simulink model "ADRC_2X2_decoupling"  (Simulink 7.6)
settings: Solver=ode45  StartTime=0.0  StopTime=300  RelTol=1e-3
values from neighbouring files (symbols this model uses):
  k = [0.28  0.2; 0.26  0.3]    [PP2013428.mat]
libraries: ADRC x2
settings Model: Creator=Administrator  LastModifiedBy=Administrator
settings DebuggingCC: AlgebraicLoopMsg=none  ArtificialAlgebraicLoopMsg=none  SolverPrmCheckMsg=none  UnknownTsInhSupMsg=none

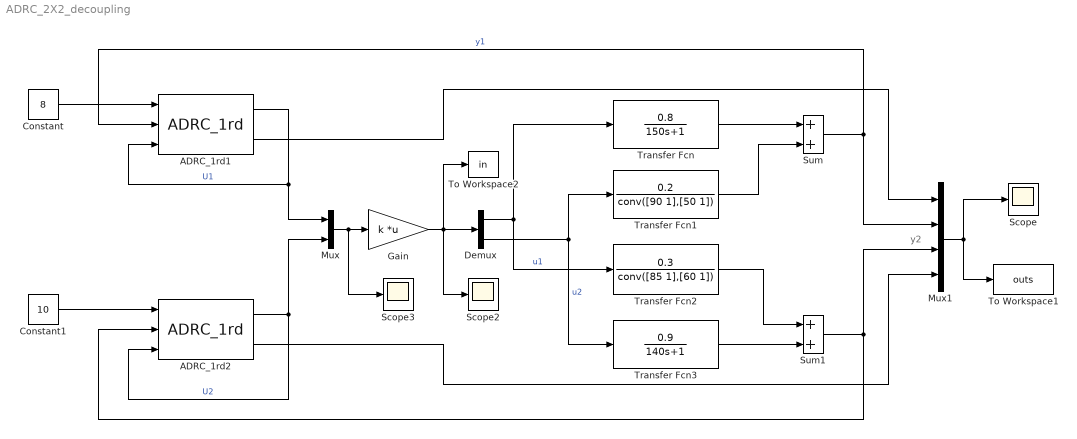
== system ADRC_2X2_decoupling ==
  note: y2
  ADRC_1rd1 : ADRC/ADRC/ADRC_1rd/ADRC_1rd  SystemSampleTime=-1  r0=0.005  h=0.1  B01=10  B02=400  r=0.3
  ADRC_1rd2 : ADRC/ADRC/ADRC_1rd/ADRC_1rd  SystemSampleTime=-1  r0=0.005  h=0.1  B01=10  B02=400  r=0.3
  Constant : Constant  Value=8
  Constant1 : Constant  Value=10
  Demux : Demux  Outputs=2
  Gain : Gain  Gain=k  Multiplication=Matrix(K*u)
  Mux : Mux  Inputs=2
  Mux1 : Mux
  Scope : Scope
      settings: TimeRange=500  YMin=7.9999  YMax=8.0002  DataFormat=Array
  Scope2 : Scope
      settings: TimeRange=500  YMax=35  SaveName=incontrol  DataFormat=Array
  Scope3 : Scope
      settings: TimeRange=500  YMin=7.9999  YMax=8.0002  SaveName=ScopeData3  DataFormat=Array
  Sum : Sum
  Sum1 : Sum
  To Workspace1 : ToWorkspace  VariableName=outs  SampleTime=1  SaveFormat=Array
  To Workspace2 : ToWorkspace  VariableName=in  SampleTime=1  SaveFormat=Array
  Transfer Fcn : TransferFcn  Numerator=0.8  Denominator=[150 1]
  Transfer Fcn1 : TransferFcn  Numerator=0.2  Denominator=conv([90 1],[50 1])
  Transfer Fcn2 : TransferFcn  Numerator=0.3  Denominator=conv([85 1],[60 1])
  Transfer Fcn3 : TransferFcn  Numerator=0.9  Denominator=[140 1]
  wires:
  Constant/1 -> ADRC_1rd1/1
  Transfer Fcn/1 -> Sum/1
  Constant1/1 -> ADRC_1rd2/1
  Mux/1 -> Gain/1, Scope3/1
  Gain/1 -> Demux/1, Scope2/1, To Workspace2/1
  ADRC_1rd1/1 -> Mux/1, ADRC_1rd1/3  "U1"
  ADRC_1rd2/1 -> Mux/2, ADRC_1rd2/3  "U2"
  Transfer Fcn3/1 -> Sum1/2
  Demux/1 -> Transfer Fcn/1, Transfer Fcn2/1  "u1"
  Demux/2 -> Transfer Fcn1/1, Transfer Fcn3/1  "u2"
  Sum/1 -> ADRC_1rd1/2, Mux1/2  "y1"
  Transfer Fcn1/1 -> Sum/2
  Transfer Fcn2/1 -> Sum1/1
  Sum1/1 -> ADRC_1rd2/2, Mux1/3
  ADRC_1rd1/2 -> Mux1/1
  Mux1/1 -> Scope/1, To Workspace1/1
  ADRC_1rd2/2 -> Mux1/4
